simulink model "FFM_Punch"  (R2017a)
settings: Solver=ode3  StartTime=0.0  StopTime=timesteps  FixedStep=data.SIM.Ts  RelTol=1e-3  EnableMultiTasking=on
values from neighbouring files (symbols this model uses):
  data =     [dakota_config.mat]
  downshift_map = data.TCU.upshift.veh_spd_default    [Simulation_results.m]
  upshift_map = data.TCU.upshift.veh_spd_default    [Simulation_results.m]
undefined symbols (not defined in the file or in its folder): air_density, Cd, DiscIntNeverNeededParam, fr_crankshaft, fr_speed_values, g, i_FD, ICE, Low_Ratio, M_Eng_Max, M_Eng_Max_Max, M_Eng_Max_Rpm, mt2m_f, mu_Roll_C0, mu_Roll_C1, mu_Roll_C2, Mv, n_Idle_Eng, Overdrive_Ratio, Re, S_eff_drag, Ts
(part 8 of 15)

== system FFM_Punch/Driver Interface/Driver Mode_pedalbased/Driver PID Error Calculation and ffwd/FirstOrderLPF1 ==
  note: Out (k) = [Tau * Out(k-1) + Ts * In(k)] / (Tau + Ts)
  note: This check is to make sure 'Tau'follows Nyquist-Shannon
      | Sampling Theorem
  Input : Inport  Tag=Controls_Lib  Description=Inp  OutDataTypeStr=single  Interpolate=off
  Tau : Inport  Tag=Controls_Lib  Description=Inp  Port=2  OutDataTypeStr=single  Interpolate=off
  b_Reset : Inport  Tag=Controls_Lib  Description=Inp  Port=3  OutDataTypeStr=boolean  Interpolate=off
  ResetValue : Inport  Tag=Controls_Lib  Description=Inp  Port=4  OutDataTypeStr=single  Interpolate=off
  AddSub2 : Sum  Tag=Controls_Lib  Description=AddSub  CollapseDim=CollapseDim  AccumDataTypeStr=single  OutMin=OutMin  OutMax=OutMax  OutDataTypeStr=single  RndMeth=Nearest  SampleTime=SampleTime  InputSameDT=on  mask(AddSub){IconShape=rectangular, Inputs=++, CollapseMode=All dimensions, CollapseDim=1, SampleTime=-1, InputSameDT=on, AccumDataTypeStr=single, OutMin=[], OutMax=[], OutDataTypeStr=single, LockScale=off, RndMeth=Nearest, SaturateOnIntegerOverflow=off}
      mask prompts: IconShape "Icon shape:"; Inputs "List of signs:"; CollapseMode "Sum over:"; CollapseDim "Dimension:"; SampleTime "Sample time (-1 for inherited):"; InputSameDT "Require all inputs to have the same data type"; AccumDataTypeStr "Accumulator data type:"; OutMin "Output minimum:"; OutMax "Output maximum:"; OutDataTypeStr "Output data type:"; LockScale "Lock data type settings against changes by the fixed-point tools"; RndMeth "Integer rounding mode:"; SaturateOnIntegerOverflow "Saturate on integer overflow"
      mask help:
      | Add or subtract inputs.  Specify one of the following:
      | a) string containing + or - for each input port, | for spacer between ports (e.g. ++|-|++)
      | b) scalar, >= 1, specifies the number of input ports to be summed.
      | When there is only one input port, add or subtract elements over all dimensions or one specified dimension
      mask Help: web([fileparts(which('Lib_built')) filesep 'hlp' filesep 'lib_AddSub' '.html'], '-helpbrowser')
      mask TypeOptions IconShape: IconShape
      mask TypeOptions Inputs: Inputs
      mask TypeOptions CollapseMode: CollapseMode
      mask TypeOptions CollapseDim: CollapseDim
      mask TypeOptions SampleTime: SampleTime
      mask TypeOptions InputSameDT: InputSameDT
      mask TypeOptions AccumDataTypeStr: AccumDataTypeStr
      mask TypeOptions OutMin: OutMin
      mask TypeOptions OutMax: OutMax
      mask TypeOptions OutDataTypeStr: OutDataTypeStr
      mask TypeOptions LockScale: LockScale
      mask TypeOptions RndMeth: RndMeth
      mask TypeOptions SaturateOnIntegerOverflow: SaturateOnIntegerOverflow
  AddSub3 : Sum  Tag=Controls_Lib  Description=AddSub  CollapseDim=CollapseDim  AccumDataTypeStr=single  OutMin=OutMin  OutMax=OutMax  OutDataTypeStr=single  RndMeth=Nearest  SampleTime=SampleTime  InputSameDT=on  mask(AddSub){IconShape=rectangular, Inputs=++, CollapseMode=All dimensions, CollapseDim=1, SampleTime=-1, InputSameDT=on, AccumDataTypeStr=single, OutMin=[], OutMax=[], OutDataTypeStr=single, LockScale=off, RndMeth=Nearest, SaturateOnIntegerOverflow=off}
      mask prompts: IconShape "Icon shape:"; Inputs "List of signs:"; CollapseMode "Sum over:"; CollapseDim "Dimension:"; SampleTime "Sample time (-1 for inherited):"; InputSameDT "Require all inputs to have the same data type"; AccumDataTypeStr "Accumulator data type:"; OutMin "Output minimum:"; OutMax "Output maximum:"; OutDataTypeStr "Output data type:"; LockScale "Lock data type settings against changes by the fixed-point tools"; RndMeth "Integer rounding mode:"; SaturateOnIntegerOverflow "Saturate on integer overflow"
      mask help:
      | Add or subtract inputs.  Specify one of the following:
      | a) string containing + or - for each input port, | for spacer between ports (e.g. ++|-|++)
      | b) scalar, >= 1, specifies the number of input ports to be summed.
      | When there is only one input port, add or subtract elements over all dimensions or one specified dimension
      mask Help: web([fileparts(which('Lib_built')) filesep 'hlp' filesep 'lib_AddSub' '.html'], '-helpbrowser')
      mask TypeOptions IconShape: IconShape
      mask TypeOptions Inputs: Inputs
      mask TypeOptions CollapseMode: CollapseMode
      mask TypeOptions CollapseDim: CollapseDim
      mask TypeOptions SampleTime: SampleTime
      mask TypeOptions InputSameDT: InputSameDT
      mask TypeOptions AccumDataTypeStr: AccumDataTypeStr
      mask TypeOptions OutMin: OutMin
      mask TypeOptions OutMax: OutMax
      mask TypeOptions OutDataTypeStr: OutDataTypeStr
      mask TypeOptions LockScale: LockScale
      mask TypeOptions RndMeth: RndMeth
      mask TypeOptions SaturateOnIntegerOverflow: SaturateOnIntegerOverflow
  Constant : Constant  Tag=Controls_Lib  Description=constant  Value=Value  OutMin=OutMin  OutMax=OutMax  OutDataTypeStr=Inherit: Inherit via back propagation  SampleTime=SampleTime  FramePeriod=FramePeriod  mask(Constant){Value=0, VectorParams1D=on, SampleTime=-1, FramePeriod=inf, OutMin=[], OutMax=[], OutDataTypeStr=Inherit: Inherit via back propagation, LockScale=off}
      mask prompts: Value "Simulink:blkprm_prompts:ConstConstValue"; VectorParams1D "Simulink:blkprm_prompts:AllSrcsVector1D"; SampleTime "Simulink:blkprm_prompts:AllSrcBlksSampleTime"; FramePeriod "Simulink:blkprm_prompts:AllSrcBlksFramePeriod"; OutMin "Simulink:blkprm_prompts:OutputDesignMin"; OutMax "Simulink:blkprm_prompts:OutputDesignMax"; OutDataTypeStr "Simulink:blkprm_prompts:OUTPUT_UNIFIEDDATATYPE"; LockScale "Simulink:blkprm_prompts:LockScale"
      mask help: Output the constant specified by the 'Constant value' parameter.
      mask Help: web([fileparts(which('Lib_built')) filesep 'hlp' filesep 'lib_constant' '.html'], '-helpbrowser')
      mask TypeOptions Value: Value
      mask TypeOptions VectorParams1D: VectorParams1D
      mask TypeOptions SampleTime: SampleTime
      mask TypeOptions FramePeriod: FramePeriod
      mask TypeOptions OutMin: OutMin
      mask TypeOptions OutMax: OutMax
      mask TypeOptions OutDataTypeStr: OutDataTypeStr
      mask TypeOptions LockScale: LockScale
      mask DialogControl ParameterTabVar0 Prompt: Main
      mask Display: disp(get_param(gcb,'Value'))
  Constant1 : Constant  Tag=Controls_Lib  Description=constant  Value=Value  OutMin=OutMin  OutMax=OutMax  OutDataTypeStr=Inherit: Inherit via back propagation  SampleTime=SampleTime  FramePeriod=FramePeriod  mask(Constant){Value=2, VectorParams1D=on, SampleTime=-1, FramePeriod=inf, OutMin=[], OutMax=[], OutDataTypeStr=Inherit: Inherit via back propagation, LockScale=off}
      mask prompts: Value "Simulink:blkprm_prompts:ConstConstValue"; VectorParams1D "Simulink:blkprm_prompts:AllSrcsVector1D"; SampleTime "Simulink:blkprm_prompts:AllSrcBlksSampleTime"; FramePeriod "Simulink:blkprm_prompts:AllSrcBlksFramePeriod"; OutMin "Simulink:blkprm_prompts:OutputDesignMin"; OutMax "Simulink:blkprm_prompts:OutputDesignMax"; OutDataTypeStr "Simulink:blkprm_prompts:OUTPUT_UNIFIEDDATATYPE"; LockScale "Simulink:blkprm_prompts:LockScale"
      mask help: Output the constant specified by the 'Constant value' parameter.
      mask Help: web([fileparts(which('Lib_built')) filesep 'hlp' filesep 'lib_constant' '.html'], '-helpbrowser')
      mask TypeOptions Value: Value
      mask TypeOptions VectorParams1D: VectorParams1D
      mask TypeOptions SampleTime: SampleTime
      mask TypeOptions FramePeriod: FramePeriod
      mask TypeOptions OutMin: OutMin
      mask TypeOptions OutMax: OutMax
      mask TypeOptions OutDataTypeStr: OutDataTypeStr
      mask TypeOptions LockScale: LockScale
      mask DialogControl ParameterTabVar0 Prompt: Main
      mask Display: disp(get_param(gcb,'Value'))
  Constant2 : Constant  Tag=Controls_Lib  Description=constant  Value=Value  OutMin=OutMin  OutMax=OutMax  OutDataTypeStr=Inherit: Inherit via back propagation  SampleTime=SampleTime  FramePeriod=FramePeriod  mask(Constant){Value=0, VectorParams1D=on, SampleTime=-1, FramePeriod=inf, OutMin=[], OutMax=[], OutDataTypeStr=Inherit: Inherit via back propagation, LockScale=off}
      mask prompts: Value "Simulink:blkprm_prompts:ConstConstValue"; VectorParams1D "Simulink:blkprm_prompts:AllSrcsVector1D"; SampleTime "Simulink:blkprm_prompts:AllSrcBlksSampleTime"; FramePeriod "Simulink:blkprm_prompts:AllSrcBlksFramePeriod"; OutMin "Simulink:blkprm_prompts:OutputDesignMin"; OutMax "Simulink:blkprm_prompts:OutputDesignMax"; OutDataTypeStr "Simulink:blkprm_prompts:OUTPUT_UNIFIEDDATATYPE"; LockScale "Simulink:blkprm_prompts:LockScale"
      mask help: Output the constant specified by the 'Constant value' parameter.
      mask Help: web([fileparts(which('Lib_built')) filesep 'hlp' filesep 'lib_constant' '.html'], '-helpbrowser')
      mask TypeOptions Value: Value
      mask TypeOptions VectorParams1D: VectorParams1D
      mask TypeOptions SampleTime: SampleTime
      mask TypeOptions FramePeriod: FramePeriod
      mask TypeOptions OutMin: OutMin
      mask TypeOptions OutMax: OutMax
      mask TypeOptions OutDataTypeStr: OutDataTypeStr
      mask TypeOptions LockScale: LockScale
      mask DialogControl ParameterTabVar0 Prompt: Main
      mask Display: disp(get_param(gcb,'Value'))
  Delay : Delay  Tag=Controls_Lib  Description=VariableDelay  RequirementInfo={} %GIDa_21d07061_4a5b_40ef_aae7_389015aa671c  DelayLength=DelayLength  DelayLengthUpperLimit=DelayLengthUpperLimit  InitialConditionSource=Input port  InitialCondition=InitialCondition  SampleTime=SampleTime  mask(Delay){DelayLengthSource=Dialog, DelayLength=1, DelayLengthUpperLimit=100, InitialConditionSource=Input port, InitialCondition=0.0, ExternalReset=None, PreventDirectFeedthrough=off, DiagnosticForOutOfRangeDelayLength=None, RemoveProtectionDelayLength=off, InputProcessing=Elements as channels (sample based), UseCircularBuffer=off, SampleTime=-1, StateName=, StateMustResolveToSignalObject=off, CodeGenStateStorageClass=Auto, CodeGenStateStorageTypeQualifier=}
      mask prompts: DelayLengthSource "Delay length source:"; DelayLength "Delay length:"; DelayLengthUpperLimit "Delay upper limit:"; InitialConditionSource "Initial condition source:"; InitialCondition "Initial condition:"; ExternalReset "External reset:"; PreventDirectFeedthrough "Prevent direct feedthrough by increasing delay length to lower limit"; DiagnosticForOutOfRangeDelayLength "Diagnostic for out-of-range delay length:"; RemoveProtectionDelayLength "Remove protection against out-of-range delay length in generated code"; InputProcessing "Input processing:"; UseCircularBuffer "Use circular buffer for state"; SampleTime "Sample time (-1 for inherited):"; StateName "State name:"; StateMustResolveToSignalObject "State name must resolve to Simulink signal object"; CodeGenStateStorageClass "Code generation storage class:"; CodeGenStateStorageTypeQualifier "Code generation storage type qualifier:"
      mask help: Delay input by a fixed or variable number of samples. The initial output of the delay block is specified by the external input x0.
      settings: InputPortMap=u0,p4
      mask Help: web([fileparts(which('Lib_discrete')) filesep 'hlp' filesep 'lib_Delay.html'], '-helpbrowser')
      mask TypeOptions DelayLengthSource: DelayLengthSource
      mask TypeOptions DelayLength: DelayLength
      mask TypeOptions DelayLengthUpperLimit: DelayLengthUpperLimit
      mask TypeOptions InitialConditionSource: InitialConditionSource
      mask TypeOptions InitialCondition: InitialCondition
      mask TypeOptions ExternalReset: ExternalReset
      mask TypeOptions PreventDirectFeedthrough: PreventDirectFeedthrough
      mask TypeOptions DiagnosticForOutOfRangeDelayLength: DiagnosticForOutOfRangeDelayLength
      mask TypeOptions RemoveProtectionDelayLength: RemoveProtectionDelayLength
      mask TypeOptions InputProcessing: InputProcessing
      mask TypeOptions UseCircularBuffer: UseCircularBuffer
      mask TypeOptions SampleTime: SampleTime
      mask TypeOptions StateName: StateName
      mask TypeOptions StateMustResolveToSignalObject: StateMustResolveToSignalObject
      mask TypeOptions CodeGenStateStorageClass: CodeGenStateStorageClass
      mask TypeOptions CodeGenStateStorageTypeQualifier: CodeGenStateStorageTypeQualifier
  IC : InitialCondition  Value=0
  MinMax : MinMax  Tag=Controls_Lib  Description=MinMax  Function=max  Inputs=Inputs  OutMin=OutMin  OutMax=OutMax  OutDataTypeStr=single  RndMeth=Zero  SampleTime=SampleTime  InputSameDT=on  mask(MinMax){Function=max, Inputs=2, ZeroCross=on, SampleTime=-1, InputSameDT=on, OutMin=[], OutMax=[], OutDataTypeStr=single, LockScale=off, RndMeth=Zero, SaturateOnIntegerOverflow=off}
      mask prompts: Inputs "Number of input ports:"; ZeroCross "Enable zero-crossing detection"; SampleTime "Sample time (-1 for inherited):"; InputSameDT "Require all inputs to have the same data type"; OutMin "Output minimum:"; OutMax "Output maximum:"; OutDataTypeStr "Output data type:"; LockScale "Lock output data type setting against changes by the fixed-point tools"; RndMeth "Integer rounding mode:"; SaturateOnIntegerOverflow "Saturate on integer overflow"
      mask help: Output min or max of input. For a single input, operators are applied across the input vector. For multiple inputs, operators are applied across the inputs.
      mask Help: web([fileparts(which('Lib_built')) filesep 'hlp' filesep 'lib_MinMax' '.html'], '-helpbrowser')
      mask TypeOptions Function: Function
      mask TypeOptions Inputs: Inputs
      mask TypeOptions ZeroCross: ZeroCross
      mask TypeOptions SampleTime: SampleTime
      mask TypeOptions InputSameDT: InputSameDT
      mask TypeOptions OutMin: OutMin
      mask TypeOptions OutMax: OutMax
      mask TypeOptions OutDataTypeStr: OutDataTypeStr
      mask TypeOptions LockScale: LockScale
      mask TypeOptions RndMeth: RndMeth
      mask TypeOptions SaturateOnIntegerOverflow: SaturateOnIntegerOverflow
  MulDiv : Product  Tag=Controls_Lib  Description=MulDiv  Inputs=**  CollapseDim=CollapseDim  OutMin=OutMin  OutMax=OutMax  OutDataTypeStr=single  SampleTime=SampleTime  InputSameDT=on  mask(MulDiv){Inputs=**, Multiplication=Element-wise(.*), CollapseMode=All dimensions, CollapseDim=1, SampleTime=-1, InputSameDT=on, OutMin=[], OutMax=[], OutDataTypeStr=single, LockScale=off, RndMeth=Floor, SaturateOnIntegerOverflow=off}
      mask prompts: Inputs "Number of inputs:"; CollapseMode "Multiply over:"; CollapseDim "Dimension:"; SampleTime "Sample time (-1 for inherited):"; InputSameDT "Require all inputs to have the same data type"; OutMin "Output minimum:"; OutMax "Output maximum:"; OutDataTypeStr "Output data type:"; LockScale "Lock output data type setting against changes by the fixed-point tools"; RndMeth "Integer rounding mode:"; SaturateOnIntegerOverflow "Saturate on integer overflow"
      mask help:
      | Multiply or divide inputs element-wise. Specify one of the following:
      |  a) * or / for each input port. For example, **/* performs the operation 'u1*u2/u3*u4'.
      |  b) scalar specifies the number of input ports to be multiplied.
      | If there is only one input port and the Multiplication parameter is set to Element-wise(.*), a single * or / collapses the input signal using the specified operation.
      mask Help: web([fileparts(which('Lib_built')) filesep 'hlp' filesep 'lib_MulDiv' '.html'], '-helpbrowser')
      mask TypeOptions Inputs: Inputs
      mask TypeOptions Multiplication: Multiplication
      mask TypeOptions CollapseMode: CollapseMode
      mask TypeOptions CollapseDim: CollapseDim
      mask TypeOptions SampleTime: SampleTime
      mask TypeOptions InputSameDT: InputSameDT
      mask TypeOptions OutMin: OutMin
      mask TypeOptions OutMax: OutMax
      mask TypeOptions OutDataTypeStr: OutDataTypeStr
      mask TypeOptions LockScale: LockScale
      mask TypeOptions RndMeth: RndMeth
      mask TypeOptions SaturateOnIntegerOverflow: SaturateOnIntegerOverflow
  MulDiv1 : Product  Tag=Controls_Lib  Description=MulDiv  Inputs=*/  CollapseDim=CollapseDim  OutMin=OutMin  OutMax=OutMax  OutDataTypeStr=single  SampleTime=SampleTime  InputSameDT=on  mask(MulDiv){Inputs=*/, Multiplication=Element-wise(.*), CollapseMode=All dimensions, CollapseDim=1, SampleTime=-1, InputSameDT=on, OutMin=[], OutMax=[], OutDataTypeStr=single, LockScale=off, RndMeth=Floor, SaturateOnIntegerOverflow=off}
      mask prompts: Inputs "Number of inputs:"; CollapseMode "Multiply over:"; CollapseDim "Dimension:"; SampleTime "Sample time (-1 for inherited):"; InputSameDT "Require all inputs to have the same data type"; OutMin "Output minimum:"; OutMax "Output maximum:"; OutDataTypeStr "Output data type:"; LockScale "Lock output data type setting against changes by the fixed-point tools"; RndMeth "Integer rounding mode:"; SaturateOnIntegerOverflow "Saturate on integer overflow"
      mask help:
      | Multiply or divide inputs element-wise. Specify one of the following:
      |  a) * or / for each input port. For example, **/* performs the operation 'u1*u2/u3*u4'.
      |  b) scalar specifies the number of input ports to be multiplied.
      | If there is only one input port and the Multiplication parameter is set to Element-wise(.*), a single * or / collapses the input signal using the specified operation.
      mask Help: web([fileparts(which('Lib_built')) filesep 'hlp' filesep 'lib_MulDiv' '.html'], '-helpbrowser')
      mask TypeOptions Inputs: Inputs
      mask TypeOptions Multiplication: Multiplication
      mask TypeOptions CollapseMode: CollapseMode
      mask TypeOptions CollapseDim: CollapseDim
      mask TypeOptions SampleTime: SampleTime
      mask TypeOptions InputSameDT: InputSameDT
      mask TypeOptions OutMin: OutMin
      mask TypeOptions OutMax: OutMax
      mask TypeOptions OutDataTypeStr: OutDataTypeStr
      mask TypeOptions LockScale: LockScale
      mask TypeOptions RndMeth: RndMeth
      mask TypeOptions SaturateOnIntegerOverflow: SaturateOnIntegerOverflow
  MulDiv4 : Product  Tag=Controls_Lib  Description=MulDiv  Inputs=**  CollapseDim=CollapseDim  OutMin=OutMin  OutMax=OutMax  OutDataTypeStr=single  SampleTime=SampleTime  InputSameDT=on  mask(MulDiv){Inputs=**, Multiplication=Element-wise(.*), CollapseMode=All dimensions, CollapseDim=1, SampleTime=-1, InputSameDT=on, OutMin=[], OutMax=[], OutDataTypeStr=single, LockScale=off, RndMeth=Floor, SaturateOnIntegerOverflow=off}
      mask prompts: Inputs "Number of inputs:"; CollapseMode "Multiply over:"; CollapseDim "Dimension:"; SampleTime "Sample time (-1 for inherited):"; InputSameDT "Require all inputs to have the same data type"; OutMin "Output minimum:"; OutMax "Output maximum:"; OutDataTypeStr "Output data type:"; LockScale "Lock output data type setting against changes by the fixed-point tools"; RndMeth "Integer rounding mode:"; SaturateOnIntegerOverflow "Saturate on integer overflow"
      mask help:
      | Multiply or divide inputs element-wise. Specify one of the following:
      |  a) * or / for each input port. For example, **/* performs the operation 'u1*u2/u3*u4'.
      |  b) scalar specifies the number of input ports to be multiplied.
      | If there is only one input port and the Multiplication parameter is set to Element-wise(.*), a single * or / collapses the input signal using the specified operation.
      mask Help: web([fileparts(which('Lib_built')) filesep 'hlp' filesep 'lib_MulDiv' '.html'], '-helpbrowser')
      mask TypeOptions Inputs: Inputs
      mask TypeOptions Multiplication: Multiplication
      mask TypeOptions CollapseMode: CollapseMode
      mask TypeOptions CollapseDim: CollapseDim
      mask TypeOptions SampleTime: SampleTime
      mask TypeOptions InputSameDT: InputSameDT
      mask TypeOptions OutMin: OutMin
      mask TypeOptions OutMax: OutMax
      mask TypeOptions OutDataTypeStr: OutDataTypeStr
      mask TypeOptions LockScale: LockScale
      mask TypeOptions RndMeth: RndMeth
      mask TypeOptions SaturateOnIntegerOverflow: SaturateOnIntegerOverflow
  MulDiv5 : Product  Tag=Controls_Lib  Description=MulDiv  Inputs=**  CollapseDim=CollapseDim  OutMin=OutMin  OutMax=OutMax  OutDataTypeStr=single  SampleTime=SampleTime  InputSameDT=on  mask(MulDiv){Inputs=**, Multiplication=Element-wise(.*), CollapseMode=All dimensions, CollapseDim=1, SampleTime=-1, InputSameDT=on, OutMin=[], OutMax=[], OutDataTypeStr=single, LockScale=off, RndMeth=Floor, SaturateOnIntegerOverflow=off}
      mask prompts: Inputs "Number of inputs:"; CollapseMode "Multiply over:"; CollapseDim "Dimension:"; SampleTime "Sample time (-1 for inherited):"; InputSameDT "Require all inputs to have the same data type"; OutMin "Output minimum:"; OutMax "Output maximum:"; OutDataTypeStr "Output data type:"; LockScale "Lock output data type setting against changes by the fixed-point tools"; RndMeth "Integer rounding mode:"; SaturateOnIntegerOverflow "Saturate on integer overflow"
      mask help:
      | Multiply or divide inputs element-wise. Specify one of the following:
      |  a) * or / for each input port. For example, **/* performs the operation 'u1*u2/u3*u4'.
      |  b) scalar specifies the number of input ports to be multiplied.
      | If there is only one input port and the Multiplication parameter is set to Element-wise(.*), a single * or / collapses the input signal using the specified operation.
      mask Help: web([fileparts(which('Lib_built')) filesep 'hlp' filesep 'lib_MulDiv' '.html'], '-helpbrowser')
      mask TypeOptions Inputs: Inputs
      mask TypeOptions Multiplication: Multiplication
      mask TypeOptions CollapseMode: CollapseMode
      mask TypeOptions CollapseDim: CollapseDim
      mask TypeOptions SampleTime: SampleTime
      mask TypeOptions InputSameDT: InputSameDT
      mask TypeOptions OutMin: OutMin
      mask TypeOptions OutMax: OutMax
      mask TypeOptions OutDataTypeStr: OutDataTypeStr
      mask TypeOptions LockScale: LockScale
      mask TypeOptions RndMeth: RndMeth
      mask TypeOptions SaturateOnIntegerOverflow: SaturateOnIntegerOverflow
  RelationalOperator : RelationalOperator  Tag=Controls_Lib  Description=RelationalOperator  Operator=>  OutDataTypeStr=boolean  SampleTime=SampleTime  RndMeth=Nearest  InputSameDT=on  mask(Relational operator){Operator=>, ZeroCross=on, SampleTime=-1, InputSameDT=on, OutDataTypeStr=boolean}
      mask prompts: Operator "Relational operator:"; ZeroCross "Enable zero-crossing detection"; SampleTime "Sample time (-1 for inherited):"; InputSameDT "Require all inputs to have the same data type"; OutDataTypeStr "Output data type:"
      mask help: Applies the selected relational operator to the inputs and outputs the result. The top (or left) input corresponds to the first operand.
      mask Help: web([fileparts(which('Lib_built')) filesep 'hlp' filesep 'lib_Relational' '.html'], '-helpbrowser')
      mask TypeOptions Operator: Operator
      mask TypeOptions ZeroCross: ZeroCross
      mask TypeOptions SampleTime: SampleTime
      mask TypeOptions InputSameDT: InputSameDT
      mask TypeOptions OutDataTypeStr: OutDataTypeStr
  Switch : Switch  Tag=Controls_Lib  Description=Switch  Criteria=u2 ~= 0  Threshold=Threshold  OutMin=OutMin  OutMax=OutMax  OutDataTypeStr=Inherit: Inherit via back propagation  RndMeth=Zero  ZeroCross=off  SampleTime=SampleTime  InputSameDT=on  mask(Switch){Criteria=u2 ~= 0, Threshold=0.5, ZeroCross=off, SampleTime=-1, InputSameDT=on, OutMin=[], OutMax=[], OutDataTypeStr=Inherit: Inherit via back propagation, LockScale=off, RndMeth=Zero, SaturateOnIntegerOverflow=off, AllowDiffInputSizes=off}
      mask prompts: Criteria "Criteria for passing first input:"; ZeroCross "Enable zero-crossing detection"; SampleTime "Sample time (-1 for inherited):"; InputSameDT "Require all data port inputs to have the same data type"; OutMin "Output minimum:"; OutMax "Output maximum:"; OutDataTypeStr "Output data type:"; LockScale "Lock output data type setting against changes by the fixed-point tools"; RndMeth "Integer rounding mode:"; SaturateOnIntegerOverflow "Saturate on integer overflow"; AllowDiffInputSizes "Allow different data input sizes (Results in variable-size output signal)"
      mask help:
      | Pass through input 1 when input 2 is not equal to 0. Otherwise, pass through input 3.  The inputs are numbered top to bottom (or left to right). The input 1 pass-through criteria are input 2 not equal to 0;
      | The first and third input ports are data ports, and the second input port is the control port. The control port signal should always be a boolean signal.
      mask Help: web([fileparts(which('Lib_built')) filesep 'hlp' filesep 'lib_Switch' '.html'], '-helpbrowser')
      mask TypeOptions Criteria: Criteria
      mask TypeOptions Threshold: Threshold
      mask TypeOptions ZeroCross: ZeroCross
      mask TypeOptions SampleTime: SampleTime
      mask TypeOptions InputSameDT: InputSameDT
      mask TypeOptions OutMin: OutMin
      mask TypeOptions OutMax: OutMax
      mask TypeOptions OutDataTypeStr: OutDataTypeStr
      mask TypeOptions LockScale: LockScale
      mask TypeOptions RndMeth: RndMeth
      mask TypeOptions SaturateOnIntegerOverflow: SaturateOnIntegerOverflow
      mask TypeOptions AllowDiffInputSizes: AllowDiffInputSizes
  Switch1 : Switch  Tag=Controls_Lib  Description=Switch  Criteria=u2 ~= 0  Threshold=Threshold  OutMin=OutMin  OutMax=OutMax  OutDataTypeStr=Inherit: Inherit via back propagation  RndMeth=Zero  ZeroCross=off  SampleTime=SampleTime  InputSameDT=on  mask(Switch){Criteria=u2 ~= 0, Threshold=0.5, ZeroCross=off, SampleTime=-1, InputSameDT=on, OutMin=[], OutMax=[], OutDataTypeStr=Inherit: Inherit via back propagation, LockScale=off, RndMeth=Zero, SaturateOnIntegerOverflow=off, AllowDiffInputSizes=off}
      mask prompts: Criteria "Criteria for passing first input:"; ZeroCross "Enable zero-crossing detection"; SampleTime "Sample time (-1 for inherited):"; InputSameDT "Require all data port inputs to have the same data type"; OutMin "Output minimum:"; OutMax "Output maximum:"; OutDataTypeStr "Output data type:"; LockScale "Lock output data type setting against changes by the fixed-point tools"; RndMeth "Integer rounding mode:"; SaturateOnIntegerOverflow "Saturate on integer overflow"; AllowDiffInputSizes "Allow different data input sizes (Results in variable-size output signal)"
      mask help:
      | Pass through input 1 when input 2 is not equal to 0. Otherwise, pass through input 3.  The inputs are numbered top to bottom (or left to right). The input 1 pass-through criteria are input 2 not equal to 0;
      | The first and third input ports are data ports, and the second input port is the control port. The control port signal should always be a boolean signal.
      mask Help: web([fileparts(which('Lib_built')) filesep 'hlp' filesep 'lib_Switch' '.html'], '-helpbrowser')
      mask TypeOptions Criteria: Criteria
      mask TypeOptions Threshold: Threshold
      mask TypeOptions ZeroCross: ZeroCross
      mask TypeOptions SampleTime: SampleTime
      mask TypeOptions InputSameDT: InputSameDT
      mask TypeOptions OutMin: OutMin
      mask TypeOptions OutMax: OutMax
      mask TypeOptions OutDataTypeStr: OutDataTypeStr
      mask TypeOptions LockScale: LockScale
      mask TypeOptions RndMeth: RndMeth
      mask TypeOptions SaturateOnIntegerOverflow: SaturateOnIntegerOverflow
      mask TypeOptions AllowDiffInputSizes: AllowDiffInputSizes
  Ts : SampleTimeMath  Tag=Controls_Lib  Description=Ts  TsampMathOp=Ts Only  weightValue=weightValue  OutDataTypeStr=Inherit: Inherit via back propagation  mask(Sample time block){TsampMathOp=Ts Only, weightValue=1, TsampMathImp=Online Calculations, OutDataTypeStr=Inherit: Inherit via back propagation, RndMeth=Floor, SaturateOnIntegerOverflow=off}
      mask prompts: TsampMathOp "Operation:"; weightValue "Weight value:"; TsampMathImp "Implement using:"; OutDataTypeStr "Output data type:"; RndMeth "Integer rounding mode:"; SaturateOnIntegerOverflow "Saturate on integer overflow"
      mask help: Sample time of the input signal
      mask Help: web([fileparts(which('Lib_built')) filesep 'hlp' filesep 'lib_Ts' '.html'], '-helpbrowser')
      mask TypeOptions TsampMathOp: TsampMathOp
      mask TypeOptions weightValue: weightValue
      mask TypeOptions TsampMathImp: TsampMathImp
      mask TypeOptions OutDataTypeStr: OutDataTypeStr
      mask TypeOptions RndMeth: RndMeth
      mask TypeOptions SaturateOnIntegerOverflow: SaturateOnIntegerOverflow
  Output : Outport  OutDataTypeStr=single  InitialOutput=0
  wires:
  IC/1 -> Switch/2
  Switch1/1 -> AddSub2/1, [Tau], Ts/1
  Tau/1 -> MinMax/2, RelationalOperator/1
  Constant2/1 -> RelationalOperator/2
  RelationalOperator/1 -> Switch1/2
  MulDiv/1 -> MinMax/1
  [Ts] -> MulDiv/2
  Constant1/1 -> MulDiv/1
  MinMax/1 -> Switch1/1
  Constant/1 -> Switch1/3
  MulDiv1/1 -> Switch/3
  [TsPlusTau] -> MulDiv1/2
  AddSub3/1 -> MulDiv1/1
  MulDiv4/1 -> AddSub3/2
  MulDiv5/1 -> AddSub3/1
  [Input] -> Delay/2
  Delay/1 -> MulDiv4/2
  [Tau] -> MulDiv4/1
  [Output] -> Delay/1
  Input/1 -> MulDiv5/1, [Input]
  [Ts] -> MulDiv5/2
  Switch/1 -> [Output], Output/1
  AddSub2/1 -> [TsPlusTau]
  Ts/1 -> [Ts], AddSub2/2
  b_Reset/1 -> IC/1
  ResetValue/1 -> Switch/1

== system FFM_Punch/Driver Interface/Driver Mode_pedalbased/Driver PID Error Calculation and ffwd/Throttle_Pedal_Determination ==
  r_Overall : Inport
  Mwheel_FFWD : Inport  Port=2
  M_eng_Max : Inport  Port=3
  Constant : Constant  Tag=Controls_Lib  Description=constant  Value=Value  OutMin=OutMin  OutMax=OutMax  OutDataTypeStr=Inherit: Inherit via back propagation  SampleTime=SampleTime  FramePeriod=FramePeriod  mask(Constant){Value=0.1, VectorParams1D=on, SampleTime=-1, FramePeriod=inf, OutMin=[], OutMax=[], OutDataTypeStr=Inherit: Inherit via back propagation, LockScale=off}
      mask prompts: Value "Simulink:blkprm_prompts:ConstConstValue"; VectorParams1D "Simulink:blkprm_prompts:AllSrcsVector1D"; SampleTime "Simulink:blkprm_prompts:AllSrcBlksSampleTime"; FramePeriod "Simulink:blkprm_prompts:AllSrcBlksFramePeriod"; OutMin "Simulink:blkprm_prompts:OutputDesignMin"; OutMax "Simulink:blkprm_prompts:OutputDesignMax"; OutDataTypeStr "Simulink:blkprm_prompts:OUTPUT_UNIFIEDDATATYPE"; LockScale "Simulink:blkprm_prompts:LockScale"
      mask help: Output the constant specified by the 'Constant value' parameter.
      mask Help: web([fileparts(which('Lib_built')) filesep 'hlp' filesep 'lib_constant' '.html'], '-helpbrowser')
      mask TypeOptions Value: Value
      mask TypeOptions VectorParams1D: VectorParams1D
      mask TypeOptions SampleTime: SampleTime
      mask TypeOptions FramePeriod: FramePeriod
      mask TypeOptions OutMin: OutMin
      mask TypeOptions OutMax: OutMax
      mask TypeOptions OutDataTypeStr: OutDataTypeStr
      mask TypeOptions LockScale: LockScale
      mask DialogControl ParameterTabVar0 Prompt: Main
      mask Display: disp(get_param(gcb,'Value'))
  Constant1 : Constant  Value=-100  OutDataTypeStr=single
  Constant2 : Constant  Tag=Controls_Lib  Description=constant  Value=Value  OutMin=OutMin  OutMax=OutMax  OutDataTypeStr=Inherit: Inherit via back propagation  SampleTime=SampleTime  FramePeriod=FramePeriod  mask(Constant){Value=0, VectorParams1D=on, SampleTime=-1, FramePeriod=inf, OutMin=[], OutMax=[], OutDataTypeStr=Inherit: Inherit via back propagation, LockScale=off}
      mask prompts: Value "Simulink:blkprm_prompts:ConstConstValue"; VectorParams1D "Simulink:blkprm_prompts:AllSrcsVector1D"; SampleTime "Simulink:blkprm_prompts:AllSrcBlksSampleTime"; FramePeriod "Simulink:blkprm_prompts:AllSrcBlksFramePeriod"; OutMin "Simulink:blkprm_prompts:OutputDesignMin"; OutMax "Simulink:blkprm_prompts:OutputDesignMax"; OutDataTypeStr "Simulink:blkprm_prompts:OUTPUT_UNIFIEDDATATYPE"; LockScale "Simulink:blkprm_prompts:LockScale"
      mask help: Output the constant specified by the 'Constant value' parameter.
      mask Help: web([fileparts(which('Lib_built')) filesep 'hlp' filesep 'lib_constant' '.html'], '-helpbrowser')
      mask TypeOptions Value: Value
      mask TypeOptions VectorParams1D: VectorParams1D
      mask TypeOptions SampleTime: SampleTime
      mask TypeOptions FramePeriod: FramePeriod
      mask TypeOptions OutMin: OutMin
      mask TypeOptions OutMax: OutMax
      mask TypeOptions OutDataTypeStr: OutDataTypeStr
      mask TypeOptions LockScale: LockScale
      mask DialogControl ParameterTabVar0 Prompt: Main
      mask Display: disp(get_param(gcb,'Value'))
  Constant3 : Constant  Tag=Controls_Lib  Description=constant  Value=Value  OutMin=OutMin  OutMax=OutMax  OutDataTypeStr=Inherit: Inherit via back propagation  SampleTime=SampleTime  FramePeriod=FramePeriod  mask(Constant){Value=2, VectorParams1D=on, SampleTime=-1, FramePeriod=inf, OutMin=[], OutMax=[], OutDataTypeStr=Inherit: Inherit via back propagation, LockScale=off}
      mask prompts: Value "Simulink:blkprm_prompts:ConstConstValue"; VectorParams1D "Simulink:blkprm_prompts:AllSrcsVector1D"; SampleTime "Simulink:blkprm_prompts:AllSrcBlksSampleTime"; FramePeriod "Simulink:blkprm_prompts:AllSrcBlksFramePeriod"; OutMin "Simulink:blkprm_prompts:OutputDesignMin"; OutMax "Simulink:blkprm_prompts:OutputDesignMax"; OutDataTypeStr "Simulink:blkprm_prompts:OUTPUT_UNIFIEDDATATYPE"; LockScale "Simulink:blkprm_prompts:LockScale"
      mask help: Output the constant specified by the 'Constant value' parameter.
      mask Help: web([fileparts(which('Lib_built')) filesep 'hlp' filesep 'lib_constant' '.html'], '-helpbrowser')
      mask TypeOptions Value: Value
      mask TypeOptions VectorParams1D: VectorParams1D
      mask TypeOptions SampleTime: SampleTime
      mask TypeOptions FramePeriod: FramePeriod
      mask TypeOptions OutMin: OutMin
      mask TypeOptions OutMax: OutMax
      mask TypeOptions OutDataTypeStr: OutDataTypeStr
      mask TypeOptions LockScale: LockScale
      mask DialogControl ParameterTabVar0 Prompt: Main
      mask Display: disp(get_param(gcb,'Value'))
  Constant4 : Constant  Value=100  OutDataTypeStr=single
  Constant5 : Constant  Tag=Controls_Lib  Description=constant  Value=Value  OutMin=OutMin  OutMax=OutMax  OutDataTypeStr=Inherit: Inherit via back propagation  SampleTime=SampleTime  FramePeriod=FramePeriod  mask(Constant){Value=0, VectorParams1D=on, SampleTime=-1, FramePeriod=inf, OutMin=[], OutMax=[], OutDataTypeStr=Inherit: Inherit via back propagation, LockScale=off}
      mask prompts: Value "Simulink:blkprm_prompts:ConstConstValue"; VectorParams1D "Simulink:blkprm_prompts:AllSrcsVector1D"; SampleTime "Simulink:blkprm_prompts:AllSrcBlksSampleTime"; FramePeriod "Simulink:blkprm_prompts:AllSrcBlksFramePeriod"; OutMin "Simulink:blkprm_prompts:OutputDesignMin"; OutMax "Simulink:blkprm_prompts:OutputDesignMax"; OutDataTypeStr "Simulink:blkprm_prompts:OUTPUT_UNIFIEDDATATYPE"; LockScale "Simulink:blkprm_prompts:LockScale"
      mask help: Output the constant specified by the 'Constant value' parameter.
      mask Help: web([fileparts(which('Lib_built')) filesep 'hlp' filesep 'lib_constant' '.html'], '-helpbrowser')
      mask TypeOptions Value: Value
      mask TypeOptions VectorParams1D: VectorParams1D
      mask TypeOptions SampleTime: SampleTime
      mask TypeOptions FramePeriod: FramePeriod
      mask TypeOptions OutMin: OutMin
      mask TypeOptions OutMax: OutMax
      mask TypeOptions OutDataTypeStr: OutDataTypeStr
      mask TypeOptions LockScale: LockScale
      mask DialogControl ParameterTabVar0 Prompt: Main
      mask Display: disp(get_param(gcb,'Value'))
  FirstOrderLPF1 : Subsystem  Tag=Controls_Lib  Description=FirstOrderLowPassFilter  RTWFcnName=Derivative_1_intial  mask(First Order Low Pass Filter){}
      mask help:
      | The First Order Low Pass Filter allows signals with a frequency lower than a certain cutoff frequency (fc) to pass through the block and attenuates signals with frequencies higher than the cutoff frequency (fc or wc).
      |
      | Inputs:
      | Input        : Signal to be Filtered
      | Tau          : Filter Time Constant (1/2*pi*fc) in Seconds defined externally
      |                  by user
      | b_Reset    : Initialization flag can be used for
      |                   controlling the filter initialization
      |                   with a non-zero initial condition “ResetValue”
      |                   When b_Reset == TRUE → Out(k)=ResetValue defined externally by
      |                   user
      | ResetValue : Filter Initial Condition defined externally by user
      |
      | Output :
      | Output : Filter Output
      |
      | Notes :
      | 1. Filter time constant should be selected such that the cut-off
      |     frequency (fc)is higher than the bandwidth of the control system.
      | 2. At First sample the b_Reset should be FALSE.
      settings: RTWFileNameOpts=Use function name
      mask Help: web([fileparts(which('Lib_discrete')) filesep 'hlp' filesep 'lib_FirstOrderLPF.html'], '-helpbrowser')
      mask Display: disp('First order\nLow Pass\nFilter');
  MinMax : MinMax  Tag=Controls_Lib  Description=MinMax  Function=max  Inputs=Inputs  OutMin=OutMin  OutMax=OutMax  OutDataTypeStr=single  RndMeth=Zero  SampleTime=SampleTime  InputSameDT=on  mask(MinMax){Function=max, Inputs=2, ZeroCross=on, SampleTime=-1, InputSameDT=on, OutMin=[], OutMax=[], OutDataTypeStr=single, LockScale=off, RndMeth=Zero, SaturateOnIntegerOverflow=off}
      mask prompts: Inputs "Number of input ports:"; ZeroCross "Enable zero-crossing detection"; SampleTime "Sample time (-1 for inherited):"; InputSameDT "Require all inputs to have the same data type"; OutMin "Output minimum:"; OutMax "Output maximum:"; OutDataTypeStr "Output data type:"; LockScale "Lock output data type setting against changes by the fixed-point tools"; RndMeth "Integer rounding mode:"; SaturateOnIntegerOverflow "Saturate on integer overflow"
      mask help: Output min or max of input. For a single input, operators are applied across the input vector. For multiple inputs, operators are applied across the inputs.
      mask Help: web([fileparts(which('Lib_built')) filesep 'hlp' filesep 'lib_MinMax' '.html'], '-helpbrowser')
      mask TypeOptions Function: Function
      mask TypeOptions Inputs: Inputs
      mask TypeOptions ZeroCross: ZeroCross
      mask TypeOptions SampleTime: SampleTime
      mask TypeOptions InputSameDT: InputSameDT
      mask TypeOptions OutMin: OutMin
      mask TypeOptions OutMax: OutMax
      mask TypeOptions OutDataTypeStr: OutDataTypeStr
      mask TypeOptions LockScale: LockScale
      mask TypeOptions RndMeth: RndMeth
      mask TypeOptions SaturateOnIntegerOverflow: SaturateOnIntegerOverflow
  Percentage : Gain  Gain=100
  Product : Product  Inputs=*/  RndMeth=Zero
  Product1 : Product  Inputs=*/  SaturateOnIntegerOverflow=on  RndMeth=Zero  InputSameDT=on  OutDataTypeStr=Inherit: Same as first input
  Saturation1 : Subsystem  Tag=Controls_Lib  Description=SaturationCheck  mask(Saturation){}
      mask help:
      | The saturation block will limit range of input signal.
      | Output will be equal to upper limit when input is above than upper limit and equal to lower limit when input is below than lower limit.
      | A flag will be set, when the block output is limited.
      |
      | Inputs:
      | UL     : Upper Limit defined externally by user
      | Input : Input coming to the Saturation block
      | LL     : Lower Limit defined externally by user
      |
      | Outputs:
      | Output                : Output of Saturation block
      | b_OutpSaturation : Flag to indicate Input is Saturated
      |
      | Note : Upper Limit should be greater than the Lower Limit
      mask Help: web([fileparts(which('Lib_discontinuous')) filesep 'hlp' filesep 'lib_Saturation.html'], '-helpbrowser')
      mask Display: plot([0 1 2 3 4 5],[0 0 0 1 1 1],[1.5 3.5],[0.5 0.5],[2.5 2.5],[0 1])
  Saturation2 : Saturate  UpperLimit=50  LowerLimit=eps
  Saturation3 : Saturate  UpperLimit=max(data.ENG.M_eng_max)  LowerLimit=0
  Terminator : Terminator
      settings: Tag=Controls_Lib  Description=Terminator
  Perc_Throtlle_FFWD : Outport
  wires:
  Product/1 -> Saturation3/1
  Product1/1 -> Percentage/1
  [M_eng_Max] -> MinMax/1  "Meng_max"
  Saturation1/2(b_OutpSaturated) -> Terminator/1
  Constant1/1 -> Saturation1/3(LL)
  Constant4/1 -> Saturation1/1(UL)
  [r_Overall] -> Saturation2/1
  Saturation2/1 -> Product/2
  r_Overall/1 -> [r_Overall]
  Mwheel_FFWD/1 -> [Mwheel_FFWD]
  [Mwheel_FFWD] -> Product/1
  Saturation3/1 -> Product1/1
  M_eng_Max/1 -> [M_eng_Max]
  Constant/1 -> MinMax/2
  MinMax/1 -> Product1/2
  Percentage/1 -> Saturation1/2(Input)
  Saturation1/1(Output) -> FirstOrderLPF1/1(Input)
  Constant3/1 -> FirstOrderLPF1/2(Tau)
  Constant2/1 -> FirstOrderLPF1/3(b_Reset)
  Constant5/1 -> FirstOrderLPF1/4(ResetValue)
  FirstOrderLPF1/1(Output) -> Perc_Throtlle_FFWD/1

== system FFM_Punch/Driver Interface/Driver Mode_pedalbased/Final PID Computation/Brake_Pedal_Determination ==
  PID_out : Inport  Tag=Controls_Lib  Description=Inp  Interpolate=off
  b_neut : Inport  Port=2
  Constant : Constant  Tag=Controls_Lib  Description=constant  Value=Value  OutMin=OutMin  OutMax=OutMax  OutDataTypeStr=single  SampleTime=SampleTime  FramePeriod=FramePeriod  mask(Constant){Value=0, VectorParams1D=on, SampleTime=-1, FramePeriod=inf, OutMin=[], OutMax=[], OutDataTypeStr=single, LockScale=off}
      mask prompts: Value "Simulink:blkprm_prompts:ConstConstValue"; VectorParams1D "Simulink:blkprm_prompts:AllSrcsVector1D"; SampleTime "Simulink:blkprm_prompts:AllSrcBlksSampleTime"; FramePeriod "Simulink:blkprm_prompts:AllSrcBlksFramePeriod"; OutMin "Simulink:blkprm_prompts:OutputDesignMin"; OutMax "Simulink:blkprm_prompts:OutputDesignMax"; OutDataTypeStr "Simulink:blkprm_prompts:OUTPUT_UNIFIEDDATATYPE"; LockScale "Simulink:blkprm_prompts:LockScale"
      mask help: Output the constant specified by the 'Constant value' parameter.
      mask Help: web([fileparts(which('Lib_built')) filesep 'hlp' filesep 'lib_constant' '.html'], '-helpbrowser')
      mask TypeOptions Value: Value
      mask TypeOptions VectorParams1D: VectorParams1D
      mask TypeOptions SampleTime: SampleTime
      mask TypeOptions FramePeriod: FramePeriod
      mask TypeOptions OutMin: OutMin
      mask TypeOptions OutMax: OutMax
      mask TypeOptions OutDataTypeStr: OutDataTypeStr
      mask TypeOptions LockScale: LockScale
      mask DialogControl ParameterTabVar0 Prompt: Main
      mask Display: disp(get_param(gcb,'Value'))
  Saturation : Saturate  UpperLimit=100  LowerLimit=0
  Saturation1 : Saturate  UpperLimit=0  LowerLimit=-100
  Switch : Switch  Tag=Controls_Lib  Description=Switch  Criteria=u2 ~= 0  Threshold=Threshold  OutMin=OutMin  OutMax=OutMax  OutDataTypeStr=Inherit: Inherit via back propagation  RndMeth=Zero  ZeroCross=off  SampleTime=SampleTime  InputSameDT=on  mask(Switch){Criteria=u2 ~= 0, Threshold=0.5, ZeroCross=off, SampleTime=-1, InputSameDT=on, OutMin=[], OutMax=[], OutDataTypeStr=Inherit: Inherit via back propagation, LockScale=off, RndMeth=Zero, SaturateOnIntegerOverflow=off, AllowDiffInputSizes=off}
      mask prompts: Criteria "Criteria for passing first input:"; ZeroCross "Enable zero-crossing detection"; SampleTime "Sample time (-1 for inherited):"; InputSameDT "Require all data port inputs to have the same data type"; OutMin "Output minimum:"; OutMax "Output maximum:"; OutDataTypeStr "Output data type:"; LockScale "Lock output data type setting against changes by the fixed-point tools"; RndMeth "Integer rounding mode:"; SaturateOnIntegerOverflow "Saturate on integer overflow"; AllowDiffInputSizes "Allow different data input sizes (Results in variable-size output signal)"
      mask help:
      | Pass through input 1 when input 2 is not equal to 0. Otherwise, pass through input 3.  The inputs are numbered top to bottom (or left to right). The input 1 pass-through criteria are input 2 not equal to 0;
      | The first and third input ports are data ports, and the second input port is the control port. The control port signal should always be a boolean signal.
      mask Help: web([fileparts(which('Lib_built')) filesep 'hlp' filesep 'lib_Switch' '.html'], '-helpbrowser')
      mask TypeOptions Criteria: Criteria
      mask TypeOptions Threshold: Threshold
      mask TypeOptions ZeroCross: ZeroCross
      mask TypeOptions SampleTime: SampleTime
      mask TypeOptions InputSameDT: InputSameDT
      mask TypeOptions OutMin: OutMin
      mask TypeOptions OutMax: OutMax
      mask TypeOptions OutDataTypeStr: OutDataTypeStr
      mask TypeOptions LockScale: LockScale
      mask TypeOptions RndMeth: RndMeth
      mask TypeOptions SaturateOnIntegerOverflow: SaturateOnIntegerOverflow
      mask TypeOptions AllowDiffInputSizes: AllowDiffInputSizes
  Driver_Brake_Request_Dcy : Outport
  Perc_Throtlle_Driv_Req_Dcy : Outport  Port=2
  wires:
  Saturation1/1 -> Switch/3  "brake_torque"
  PID_out/1 -> Saturation1/1, Saturation/1
  Saturation/1 -> Perc_Throtlle_Driv_Req_Dcy/1
  b_neut/1 -> Switch/2
  Constant/1 -> Switch/1
  Switch/1 -> Driver_Brake_Request_Dcy/1
